simulink model "M44"  (R2021b)
settings: Solver=VariableStepAuto  StartTime=0.0  StopTime=10  RelTol=1e-3
settings Model: Creator=abdul  LastModifiedBy=abdul

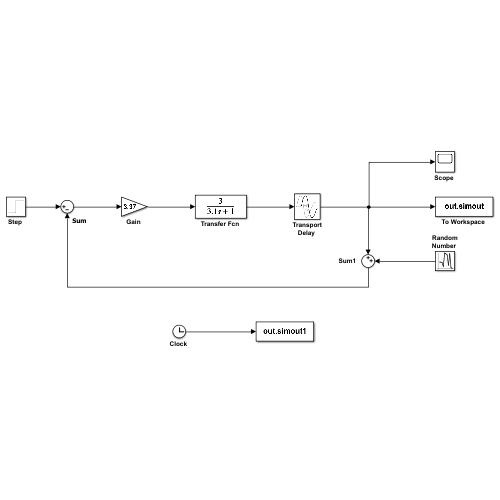
[thumbnail: Simulink's stored preview of the top-level diagram]
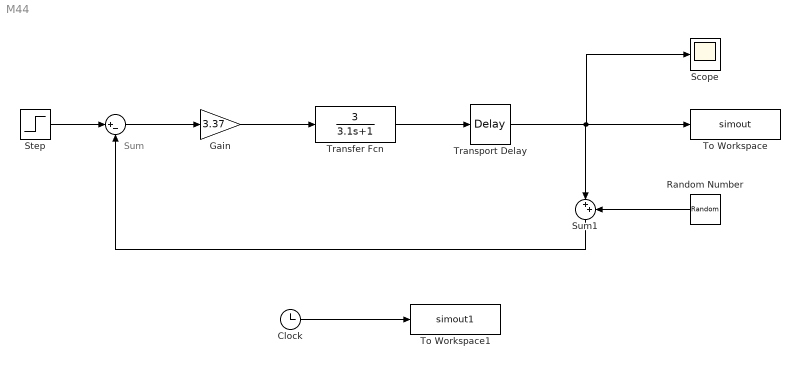
== system M44 ==
  note: Sum
  " " : Sum  Inputs=|+-
  "Clock " : Clock
  "Gain " : Gain  Gain=3.37
  "Random Number " : RandomNumber  Variance=0.5  Seed=61233  SampleTime=0
  "Scope " : Scope
  "Step " : Step  Time=0  After=30  SampleTime=0
  "Sum1 " : Sum  Inputs=|++
  "To Workspace " : ToWorkspace  VariableName=simout  SaveFormat=Timeseries  SampleTime=-1
  To Workspace1 : ToWorkspace  VariableName=simout1  SaveFormat=Timeseries  SampleTime=-1
  "Transfer Fcn " : TransferFcn  Numerator=[3]  Denominator=[3.1 1]
  "Transport Delay " : TransportDelay  DelayTime=0.15
  wires:
  "Step "/1 -> " "/1
  " "/1 -> "Gain "/1
  "Gain "/1 -> "Transfer Fcn "/1
  "Clock "/1 -> To Workspace1/1
  "Transfer Fcn "/1 -> "Transport Delay "/1
  "Transport Delay "/1 -> "To Workspace "/1, "Scope "/1, "Sum1 "/1
  "Random Number "/1 -> "Sum1 "/2
  "Sum1 "/1 -> " "/2
